simulink model "RTInductionMotorJan27"  (R2020a)
settings: Solver=FixedStepAuto  StartTime=0.0  StopTime=5  FixedStep=100e-6  RelTol=1e-3
model workspace (MAT data in the model file):
  Fe = 60
  Poles = 2
libraries: powerlib x26, simulink x4, powerlib_meascontrol x4
(part 1 of 2)
settings Model: Creator=adam_  LastModifiedBy=Yaipiti
settings SolverCC: AlgebraicLoopSolver=LineSearch
settings SFSimCC: CustomCodeUndefinedFunction=UseInterfaceOnly

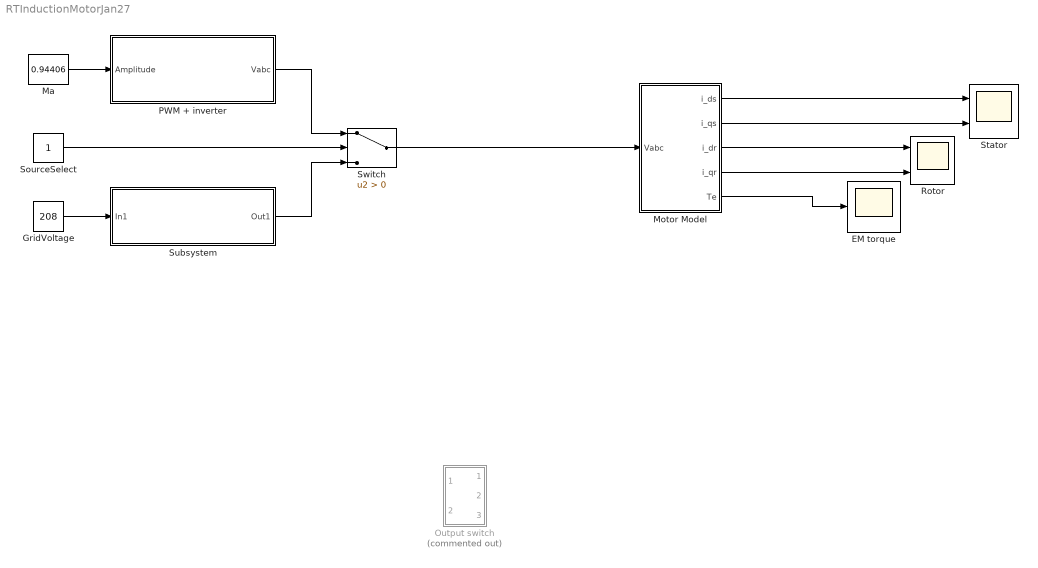
== system RTInductionMotorJan27 ==
  EM torque : Scope
  GridVoltage : Constant  Value=208
  Ma : Constant  Value=0.94406
  Motor Model : Subsystem
  Output switch : Subsystem  Commented=on
  PWM + inverter : Subsystem
  Rotor : Scope  NumInputPorts=2
  SourceSelect : Constant
  Stator : Scope  NumInputPorts=2
  Subsystem : Subsystem
  Switch : Switch  Criteria=u2 > Threshold
  wires:
  Motor Model/1(i_ds) -> Stator/1
  Motor Model/2(i_qs) -> Stator/2
  Motor Model/3(i_dr) -> Rotor/1
  Motor Model/4(i_qr) -> Rotor/2
  Motor Model/5(Te) -> EM torque/1
  Ma/1 -> PWM + inverter/1(Amplitude)
  GridVoltage/1 -> Subsystem/1(In1)
  Subsystem/1(Out1) -> Switch/3
  Switch/1 -> Motor Model/1(Vabc)
  SourceSelect/1 -> Switch/2
  PWM + inverter/1(Vabc) -> Switch/1

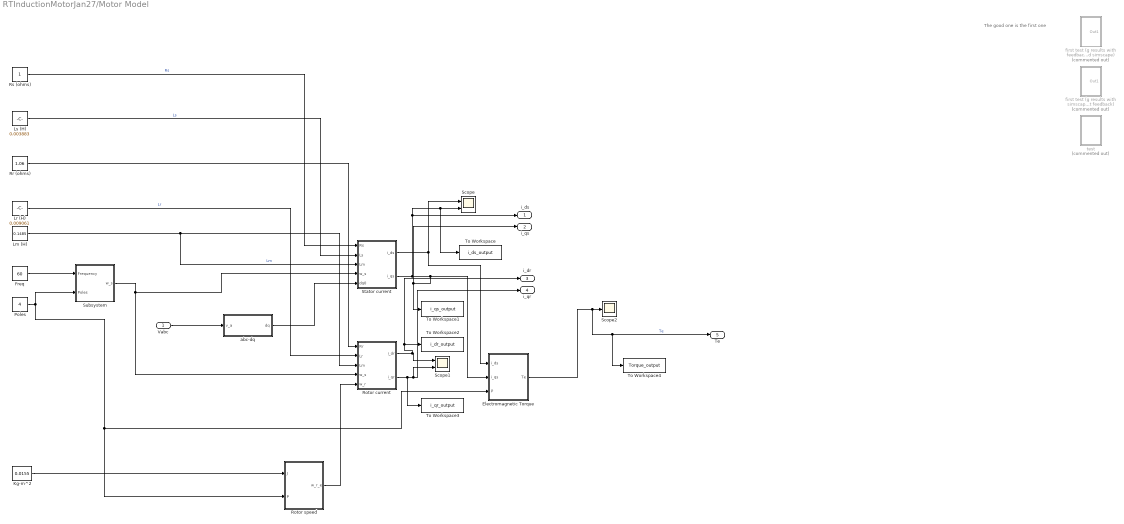
== system RTInductionMotorJan27/Motor Model ==
  note: The good one is the first one
  Vabc : Inport
  Electromagnetic Torque : Subsystem
  Freq : Constant  Value=60
  Kg-m^2 : Constant  Value=0.0155
  Lm (H) : Constant  Value=0.1485
  Lr (H) : Constant  Value=0.009061
  Ls (H) : Constant  Value=0.003883
  Poles : Constant  Value=4
  Rotor current : Subsystem
  Rotor speed : Subsystem
  Rr (ohms) : Constant  Value=1.06
  Rs (ohms) : Constant
  Scope : Scope  NumInputPorts=2
  Scope1 : Scope  NumInputPorts=2
  Scope2 : Scope
  Stator current : Subsystem
  Subsystem : Subsystem
  To Workspace : ToWorkspace  VariableName=i_ds_output  SaveFormat=Timeseries  SampleTime=-1
  To Workspace1 : ToWorkspace  VariableName=i_qs_output  SaveFormat=Timeseries  SampleTime=-1
  To Workspace2 : ToWorkspace  VariableName=i_dr_output  SaveFormat=Timeseries  SampleTime=-1
  To Workspace3 : ToWorkspace  VariableName=i_qr_output  SaveFormat=Timeseries  SampleTime=-1
  To Workspace4 : ToWorkspace  VariableName=Torque_output  SaveFormat=Timeseries  SampleTime=-1
  abc-dq : Subsystem
  first test (g results with feedback and simscape) : Subsystem  Commented=on
  first test (g results with simscape but without feedback) : Subsystem  Commented=on
  test : Subsystem  Commented=on
  i_ds : Outport
  i_qs : Outport  Port=2
  i_dr : Outport  Port=3
  i_qr : Outport  Port=4
  Te : Outport  Port=5
  wires:
  Vabc/1 -> abc-dq/1(v_a)
  Electromagnetic Torque/1(Te) -> Te/1, To Workspace4/1, Scope2/1  "Te"
  Lm (H)/1 -> Rotor current/3(Lm), Stator current/3(Lm)  "Lm"
  abc-dq/1(dq) -> Stator current/5(dq0)
  Lr (H)/1 -> Rotor current/2(Lr)  "Lr"
  Rs (ohms)/1 -> Stator current/1(Rs)  "Rs"
  Subsystem/1(w_s) -> Rotor current/4(w_s), Stator current/4(w_s)
  Kg-m^2/1 -> Rotor speed/1(J)
  Ls (H)/1 -> Stator current/2(Ls)  "Ls"
  Stator current/1(i_ds) -> Electromagnetic Torque/1(i_ds), Scope/1
  Freq/1 -> Subsystem/1(Frequency)
  Rotor speed/1(w_r_e) -> Rotor current/5(w_r)
  Rr (ohms)/1 -> Rotor current/1(Rr)
  Stator current/2(i_qs) -> To Workspace1/1, i_qs/1, Electromagnetic Torque/2(i_qs), i_ds/1, To Workspace/1, Scope/2
  Rotor current/2(i_qr) -> To Workspace3/1, i_qr/1, Scope1/2
  Poles/1 -> Subsystem/2(Poles), Rotor speed/2(P), Electromagnetic Torque/3(P)
  Rotor current/1(i_dr) -> i_dr/1, To Workspace2/1, Scope1/1

== system RTInductionMotorJan27/Output switch ==
  Signal : Inport
  Choice : Inport  Port=2
  Add : Sum  Inputs=+-
  Add1 : Sum  Inputs=+-
  Add2 : Sum  Inputs=+-
  Constant1 : Constant  Value=2
  Constant2 : Constant
  Constant3 : Constant  Value=3
  IsZero : simulink/Logic and Bit Operations/Compare To Zero  relop===  OutDataTypeStr=boolean
  IsZero1 : simulink/Logic and Bit Operations/Compare To Zero  relop===  OutDataTypeStr=boolean
  IsZero2 : simulink/Logic and Bit Operations/Compare To Zero  relop===  OutDataTypeStr=boolean
  Product : Product
  Product1 : Product
  Product2 : Product
  Out1 : Outport
  Out2 : Outport  Port=2
  Out3 : Outport  Port=3
  wires:
  Add1/1 -> IsZero1/1
  Product2/1 -> Out3/1
  Signal/1 -> Product/2, Product1/2, Product2/2
  Choice/1 -> Add2/1, Add1/1, Add/1
  IsZero2/1 -> Product2/1
  Constant1/1 -> Add/2
  Add/1 -> IsZero/1
  Add2/1 -> IsZero2/1
  Constant3/1 -> Add2/2
  IsZero/1 -> Product/1
  Constant2/1 -> Add1/2
  IsZero1/1 -> Product1/1
  Product1/1 -> Out2/1
  Product/1 -> Out1/1

== system RTInductionMotorJan27/PWM + inverter ==
  Amplitude : Inport
  Mux : Mux  Inputs=3
  Product : Product
  Product1 : Product
  Product2 : Product
  Scope : Scope
  Sine Wave : Sin  Frequency=2*pi*60  SampleTime=0
  Sine Wave1 : Sin  Frequency=2*pi*60  Phase=-2*pi/3  SampleTime=0
  Sine Wave2 : Sin  Frequency=2*pi*60  Phase=2*pi/3  SampleTime=0
  Three-phase PWM : Subsystem
  Vdc : Constant  Value=360
  inverter : Subsystem
  Vabc : Outport
  wires:
  Mux/1 -> Three-phase PWM/1(Signals)
  Three-phase PWM/1(Pulses) -> inverter/2(Pulses)
  inverter/1(Vabc) -> Scope/1, Vabc/1
  Vdc/1 -> inverter/1(Vdc)
  Sine Wave/1 -> Product/2
  Amplitude/1 -> Product2/1, Product1/1, Product/1
  Product/1 -> Mux/1
  Product2/1 -> Mux/3
  Product1/1 -> Mux/2
  Sine Wave1/1 -> Product1/2
  Sine Wave2/1 -> Product2/2

== system RTInductionMotorJan27/Subsystem ==
  In1 : Inport
  Mux : Mux  Inputs=3
  Product : Product
  Product1 : Product
  Product2 : Product
  Sine Wave : Sin  Frequency=2*pi*60  SampleTime=0
  Sine Wave1 : Sin  Frequency=2*pi*60  Phase=-2*pi/3  SampleTime=0
  Sine Wave2 : Sin  Frequency=2*pi*60  Phase=2*pi/3  SampleTime=0
  Out1 : Outport
  wires:
  Sine Wave/1 -> Product/2
  Product/1 -> Mux/1
  In1/1 -> Product2/1, Product1/1, Product/1
  Sine Wave1/1 -> Product1/2
  Sine Wave2/1 -> Product2/2
  Product2/1 -> Mux/3
  Product1/1 -> Mux/2
  Mux/1 -> Out1/1

== system RTInductionMotorJan27/Motor Model/Electromagnetic Torque ==
  i_ds : Inport
  i_qs : Inport  Port=2
  P : Inport  Port=3
  Constant : Constant  Value=3/4
  Product{,1..3} (4 alike) : Product
  Subtract : Sum  Inputs=+-
  Te : Outport  VectorParamsAs1DForOutWhenUnconnected=off
  tag scope: Te=global
  wires:
  Product3/1 -> Te/1, [Te]
  Subtract/1 -> Product3/1
  Product2/1 -> Product3/2
  Constant/1 -> Product2/2
  P/1 -> Product2/1
  Product1/1 -> Subtract/2
  Product/1 -> Subtract/1
  i_ds/1 -> Product1/2
  [flux_qs] -> Product1/1
  [flux_ds] -> Product/2
  i_qs/1 -> Product/1

== system RTInductionMotorJan27/Motor Model/Rotor current ==
  Rr : Inport
  Lr : Inport  Port=2
  Lm : Inport  Port=3
  w_s : Inport  Port=4
  w_r : Inport  Port=5
  Rotor Flux : Subsystem
  Rotor currents : Subsystem
  Subtract : Sum  Inputs=+-
  i_dr : Outport  VectorParamsAs1DForOutWhenUnconnected=off
  i_qr : Outport  Port=2  VectorParamsAs1DForOutWhenUnconnected=off
  wires:
  Subtract/1 -> Rotor Flux/2(w_s1)
  w_r/1 -> Subtract/2
  Rotor currents/2(i_qr) -> i_qr/1
  Rotor currents/1(i_dr) -> i_dr/1
  Rotor Flux/1(flux_dr) -> Rotor currents/1(flux_dr)  "flux_dr"
  Rotor Flux/2(flux_qr) -> Rotor currents/2(flus_qr)  "flux_qr"
  Lr/1 -> Rotor currents/3(Lr)
  w_s/1 -> Subtract/1
  Rr/1 -> Rotor Flux/1(Rr (Ohms))
  Lm/1 -> Rotor currents/4(Lm)

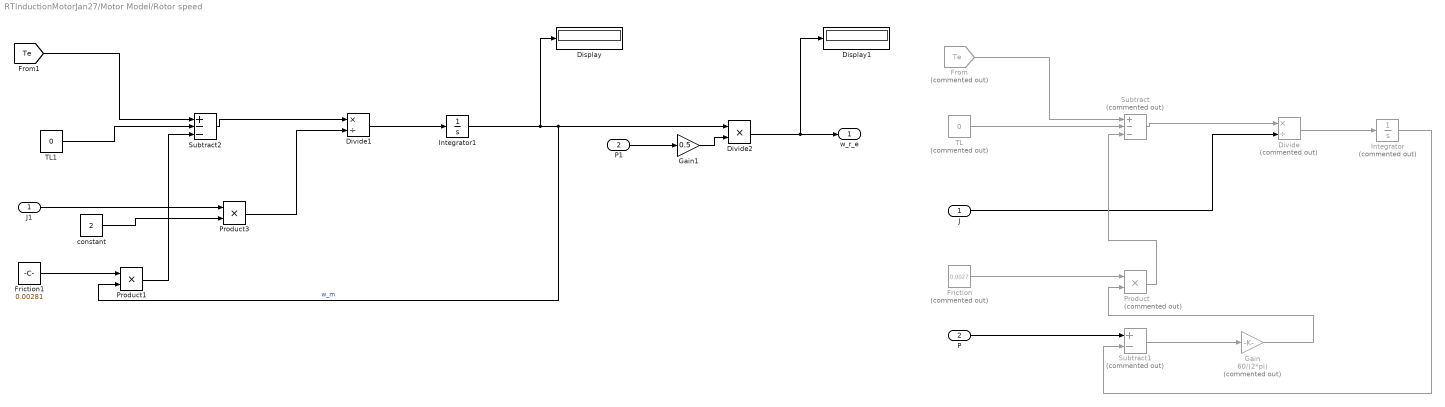
== system RTInductionMotorJan27/Motor Model/Rotor speed ==
  J : Inport
  P : Inport  Port=2
  Display : Display
  Display1 : Display
  Divide : Product  Commented=on  Inputs=*/
  Divide1 : Product  Inputs=*/
  Divide2 : Product  Inputs=**
  Friction : Constant  Commented=on  Value=0.0027
  Friction1 : Constant  Value=0.00281
  From : From  Commented=on  GotoTag=Te  TagVisibility=global
  Gain : Gain  Commented=on  Gain=60/(2*pi)
  Gain1 : Gain  Gain=0.5
  Integrator : Integrator  Commented=on
  Integrator1 : Integrator
  J1 : InportShadow
  P1 : InportShadow  Port=2
  Product : Product  Commented=on
  Product1 : Product
  Product3 : Product
  Subtract : Sum  Commented=on  Inputs=+--
  Subtract1 : Sum  Commented=on  Inputs=+-
  Subtract2 : Sum  Inputs=+--
  TL : Constant  Commented=on  Value=0
  TL1 : Constant  Value=0
  constant : Constant  Value=2
  w_r_e : Outport  VectorParamsAs1DForOutWhenUnconnected=off
  wires:
  From/1 -> Subtract/1
  TL/1 -> Subtract/2
  Subtract/1 -> Divide/1
  J/1 -> Divide/2
  Divide/1 -> Integrator/1
  Integrator/1 -> Subtract1/2
  P/1 -> Subtract1/1
  Subtract1/1 -> Gain/1
  Gain/1 -> Product/2
  Friction/1 -> Product/1
  Product/1 -> Subtract/3
  [Te] -> Subtract2/1
  Subtract2/1 -> Divide1/1
  Divide1/1 -> Integrator1/1
  TL1/1 -> Subtract2/2
  Friction1/1 -> Product1/1
  Product1/1 -> Subtract2/3
  J1/1 -> Product3/1
  constant/1 -> Product3/2
  Product3/1 -> Divide1/2
  Integrator1/1 -> Display/1, Product1/2, Divide2/1  "w_m"
  P1/1 -> Gain1/1
  Gain1/1 -> Divide2/2
  Divide2/1 -> Display1/1, w_r_e/1

== system RTInductionMotorJan27/Motor Model/Stator current ==
  Rs : Inport
  Ls : Inport  Port=2
  Lm : Inport  Port=3
  w_s : Inport  Port=4
  dq0 : Inport  Port=5
  Stator Flux : Subsystem
  Stator currents : Subsystem
  i_ds : Outport  VectorParamsAs1DForOutWhenUnconnected=off
  i_qs : Outport  Port=2  VectorParamsAs1DForOutWhenUnconnected=off
  wires:
  dq0/1 -> Stator Flux/3(dq0)
  Stator currents/2(i_qs) -> i_qs/1
  w_s/1 -> Stator Flux/2(w_s)
  Stator currents/1(i_ds) -> i_ds/1
  Lm/1 -> Stator currents/4(Lm)
  Ls/1 -> Stator currents/3(Ls)
  Rs/1 -> Stator Flux/1(Rs (Ohms))
  Stator Flux/1(flux_ds) -> Stator currents/1(flus_ds)  "flux_ds"
  Stator Flux/2(flux_qs) -> Stator currents/2(flus_qs)  "flux_qs"

== system RTInductionMotorJan27/Motor Model/Subsystem ==
  Frequency : Inport
  Poles : Inport  Port=2
  Constant : Constant  Commented=on  Value=120
  Constant1 : Constant  Commented=on  Value=2*pi
  Display : Display
  Divide2 : Product  Inputs=**/
  Frequency1 : InportShadow
  Gain : Gain  Gain=0.5
  Integrator : Integrator  Commented=on
  Poles1 : InportShadow  Port=2
  Product : Product
  Rem : Math  Commented=on  Operator=rem  SignedPower=on  SaturateOnIntegerOverflow=on
  constant1 : Constant  Value=120
  multipliy : Product  Commented=on  Inputs=**
  ns (rpm) : Product  Commented=on  Inputs=**/
  rpm to rad/s : Gain  Gain=2*pi/60
  w_s_gain : Gain  Commented=on  Gain=2*pi/60
  w_s : Outport  VectorParamsAs1DForOutWhenUnconnected=off
  wires:
  Integrator/1 -> Rem/1
  Rem/1 -> ?
  Constant1/1 -> Rem/2
  Constant/1 -> ns (rpm)/2
  Frequency/1 -> ns (rpm)/1
  Poles/1 -> multipliy/2, ns (rpm)/3
  ns (rpm)/1 -> multipliy/1
  w_s_gain/1 -> Integrator/1  "w_s"
  multipliy/1 -> w_s_gain/1
  constant1/1 -> Divide2/1
  Divide2/1 -> rpm to rad/s/1  "n_s"
  Frequency1/1 -> Divide2/2
  Poles1/1 -> Gain/1, Divide2/3
  rpm to rad/s/1 -> Display/1, Product/1
  Product/1 -> w_s/1
  Gain/1 -> Product/2

== system RTInductionMotorJan27/Motor Model/abc-dq ==
  v_a : Inport
  Add : Sum
  Constant : Constant  Value=2*pi*60
  Constant1 : Constant  Value=-pi/3
  Integrator : Integrator
  Mux3 : Mux  Inputs=2
  Mux4 : Mux  Inputs=2
  Scope2 : Scope
  Scope3 : Scope
  Vd : Fcn  Expr=sqrt(2/3)*(u(1)*cos(u(4))+u(2)*cos(u(4)-2*pi/3)+u(3)*cos(u(4)+2*pi/3))
  Vq : Fcn  Expr=-sqrt(2/3)*(u(1)*sin(u(4))+u(2)*sin(u(4)-2*pi/3)+u(3)*sin(u(4)+2*pi/3))
  dq : Outport  VectorParamsAs1DForOutWhenUnconnected=off
  wires:
  v_a/1 -> Mux3/1
  Mux3/1 -> Vd/1, Vq/1, Scope2/1
  Constant/1 -> Integrator/1
  Integrator/1 -> Add/1  "w_t"
  Constant1/1 -> Add/2
  Add/1 -> Mux3/2
  Vd/1 -> Mux4/1
  Vq/1 -> Mux4/2
  Mux4/1 -> dq/1, Scope3/1

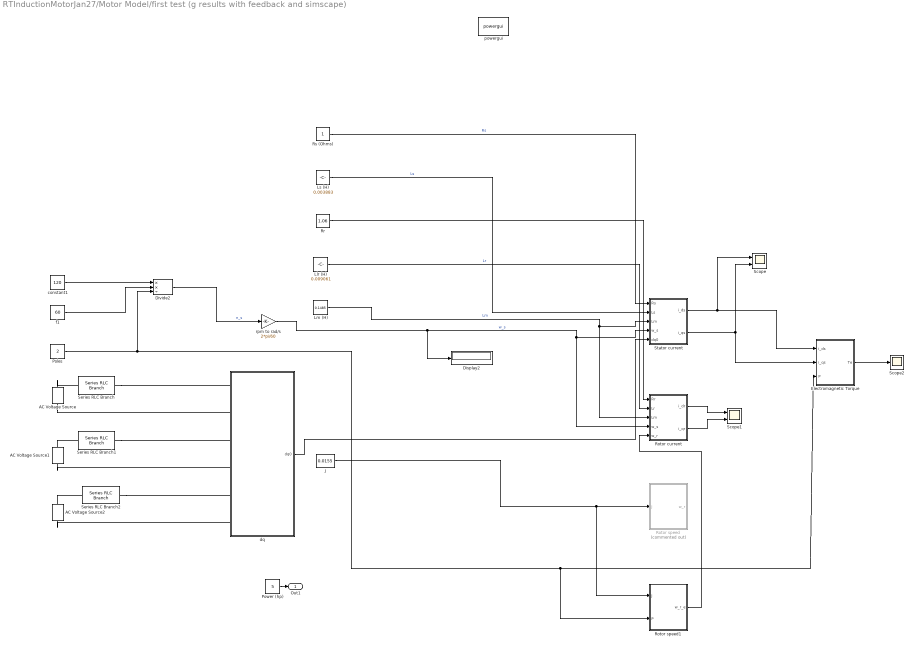
== system RTInductionMotorJan27/Motor Model/first test (g results with feedback and simscape) ==
  AC Voltage Source : powerlib/Electrical Sources/AC Voltage Source  Amplitude=340  Phase=0  Frequency=50  SampleTime=0  Measurements=Voltage  BusType=swing  Pref=10e3  Qref=0  Qmin=-inf  Qmax=+inf
  AC Voltage Source1 : powerlib/Electrical Sources/AC Voltage Source  Amplitude=340  Phase=-120  Frequency=50  SampleTime=0  Measurements=Voltage  BusType=swing  Pref=10e3  Qref=0  Qmin=-inf  Qmax=+inf
  AC Voltage Source2 : powerlib/Electrical Sources/AC Voltage Source  Amplitude=340  Phase=120  Frequency=50  SampleTime=0  Measurements=Voltage  BusType=swing  Pref=10e3  Qref=0  Qmin=-inf  Qmax=+inf
  Display2 : Display
  Divide2 : Product  Inputs=**/
  Electromagnetic Torque : Subsystem
  J : Constant  Value=0.0155
  Llr (H) : Constant  Value=0.009061
  Lm (H) : Constant  Value=0.1485
  Ls (H) : Constant  Value=0.003883
  Poles : Constant  Value=2
  Power (hp) : Constant  Value=5
  Rotor current : Subsystem
  Rotor speed : Subsystem  Commented=on
  Rotor speed1 : Subsystem
  "Rr " : Constant  Value=1.06
  Rs (Ohms) : Constant
  Scope : Scope  NumInputPorts=2
  Scope1 : Scope  NumInputPorts=2
  Scope2 : Scope
  Series RLC Branch : powerlib/Elements/Series RLC Branch  LConnTagsString=__new0  RConnTagsString=__new0  BranchType=R  Resistance=0.1  Inductance=1e-3  SetiL0=off  InitialCurrent=0  Capacitance=1e-6  Setx0=off  InitialVoltage=0  Measurements=None
  Series RLC Branch1 : powerlib/Elements/Series RLC Branch  LConnTagsString=__new0  RConnTagsString=__new0  BranchType=R  Resistance=0.1  Inductance=1e-3  SetiL0=off  InitialCurrent=0  Capacitance=1e-6  Setx0=off  InitialVoltage=0  Measurements=None
  Series RLC Branch2 : powerlib/Elements/Series RLC Branch  LConnTagsString=__new0  RConnTagsString=__new0  BranchType=R  Resistance=0.1  Inductance=1e-3  SetiL0=off  InitialCurrent=0  Capacitance=1e-6  Setx0=off  InitialVoltage=0  Measurements=None
  Stator current : Subsystem
  constant1 : Constant  Value=120
  dq : Subsystem
  f1 : Constant  Value=60
  powergui : powerlib/powergui  Priority=1  SimulationMode=Continuous  SampleTime=50e-6  frequency=60  Iterations=50  frequencyindice=50  Pbase=100e6  ErrMax=1e-4  UnitsV=kV  UnitsW=MW  buscounter=0  FunctionMessages=off  echomessages=off  EnableUseOfTLC=off  CurrentSourceSwitches=off  DisableSnubberDevices=off  DisableRonSwitches=off  DisableVfSwitches=off  DisplayEquations=off  AutomaticDiscreteSolvers=off  SolverType=Tustin/Backward Euler (TBE)  Interpol=off  ExternalGateDelay=off  methode=off  Ts=100  x0status=blocks  SPID=on  SwTol=0  HookPort=off  NonlinearTolerance=1e-4  nMaxIteration=100  ContinueOnMaxIteration=off  RestoreLinks=warning  ResistiveCurrentMeasurement=off  Frange=[0:2:500]  Ylog=off  Xlog=on  ShowGrid=off  save=off  variable=ZData  structure=0  ZoomFFT=off  StartTime=0.0  cycles=1  DisplayStyle=1  fundamental=60  FreqAxis=off  MaxFrequency=1000  frequencyindicesteady=1  RmsSteady=1  display=off
  rpm to rad/s : Gain  Gain=2*pi/60
  Out1 : Outport  VectorParamsAs1DForOutWhenUnconnected=off
  wires:
  J/1 -> Rotor speed1/1(J), Rotor speed/1(J)
  Stator current/2(i_qs) -> Scope/2, Electromagnetic Torque/2(i_qs)
  Electromagnetic Torque/1(Te) -> Scope2/1
  Rotor current/2(i_qr) -> Scope1/2
  "Rr "/1 -> Rotor current/1(Rr)
  Ls (H)/1 -> Stator current/2(Ls)  "Ls"
  rpm to rad/s/1 -> Display2/1, Rotor current/4(w_s), Stator current/4(w_s)  "w_s"
  Lm (H)/1 -> Rotor current/3(Lm), Stator current/3(Lm)  "Lm"
  Poles/1 -> Divide2/3, Rotor speed1/2(P), Electromagnetic Torque/3(P)
  Rotor current/1(i_dr) -> Scope1/1
  Stator current/1(i_ds) -> Scope/1, Electromagnetic Torque/1(i_ds)
  Llr (H)/1 -> Rotor current/2(Lr)  "Lr"
  Rs (Ohms)/1 -> Stator current/1(Rs)  "Rs"
  dq/1(dq0) -> Stator current/5(dq0)
  Power (hp)/1 -> Out1/1
  Rotor speed1/1(w_r_e) -> Rotor current/5(w_r)
  f1/1 -> Divide2/2
  constant1/1 -> Divide2/1
  Divide2/1 -> rpm to rad/s/1  "n_s"
  connections:
  AC Voltage Source/LConn1 -- dq/LConn2
  Series RLC Branch2/RConn1 -- dq/LConn5
  AC Voltage Source2/RConn1 -- Series RLC Branch2/LConn1
  AC Voltage Source1/RConn1 -- Series RLC Branch1/LConn1
  AC Voltage Source/RConn1 -- Series RLC Branch/LConn1
  AC Voltage Source2/LConn1 -- dq/LConn6
  Series RLC Branch/RConn1 -- dq/LConn1
  AC Voltage Source1/LConn1 -- dq/LConn4
  Series RLC Branch1/RConn1 -- dq/LConn3

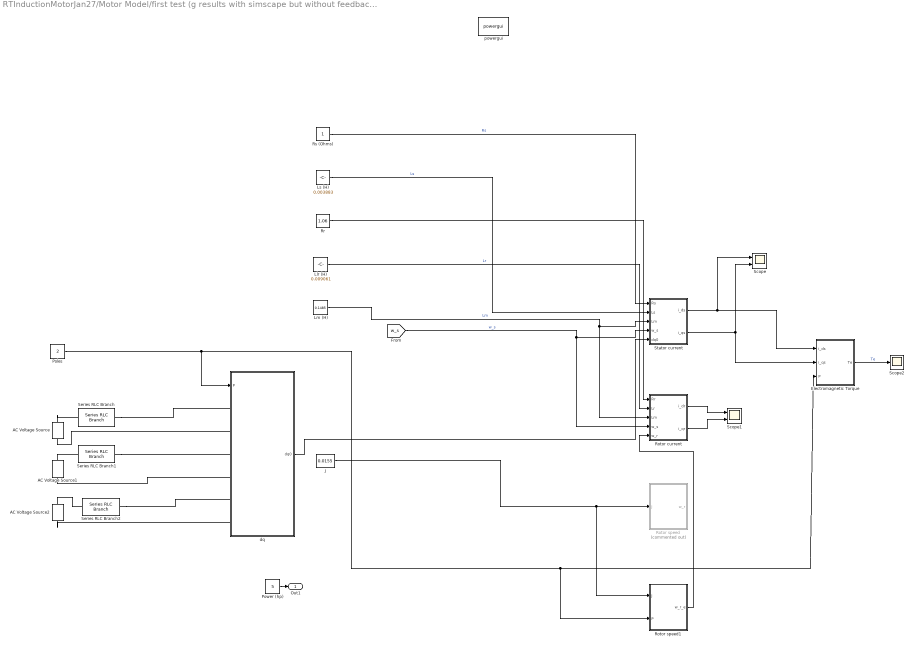
== system RTInductionMotorJan27/Motor Model/first test (g results with simscape but without feedback) ==
  AC Voltage Source : powerlib/Electrical Sources/AC Voltage Source  Amplitude=340  Phase=0  Frequency=50  SampleTime=0  Measurements=None  BusType=swing  Pref=10e3  Qref=0  Qmin=-inf  Qmax=+inf
  AC Voltage Source1 : powerlib/Electrical Sources/AC Voltage Source  Amplitude=340  Phase=-120  Frequency=50  SampleTime=0  Measurements=None  BusType=swing  Pref=10e3  Qref=0  Qmin=-inf  Qmax=+inf
  AC Voltage Source2 : powerlib/Electrical Sources/AC Voltage Source  Amplitude=340  Phase=120  Frequency=50  SampleTime=0  Measurements=None  BusType=swing  Pref=10e3  Qref=0  Qmin=-inf  Qmax=+inf
  Electromagnetic Torque : Subsystem
  J : Constant  Value=0.0155
  Llr (H) : Constant  Value=0.009061
  Lm (H) : Constant  Value=0.1485
  Ls (H) : Constant  Value=0.003883
  Poles : Constant  Value=2
  Power (hp) : Constant  Value=5
  Rotor current : Subsystem
  Rotor speed : Subsystem  Commented=on
  Rotor speed1 : Subsystem
  "Rr " : Constant  Value=1.06
  Rs (Ohms) : Constant
  Scope : Scope  NumInputPorts=2
  Scope1 : Scope  NumInputPorts=2
  Scope2 : Scope
  Series RLC Branch : powerlib/Elements/Series RLC Branch  LConnTagsString=__new0  RConnTagsString=__new0  BranchType=R  Resistance=0.1  Inductance=1e-3  SetiL0=off  InitialCurrent=0  Capacitance=1e-6  Setx0=off  InitialVoltage=0  Measurements=None
  Series RLC Branch1 : powerlib/Elements/Series RLC Branch  LConnTagsString=__new0  RConnTagsString=__new0  BranchType=R  Resistance=0.1  Inductance=1e-3  SetiL0=off  InitialCurrent=0  Capacitance=1e-6  Setx0=off  InitialVoltage=0  Measurements=None
  Series RLC Branch2 : powerlib/Elements/Series RLC Branch  LConnTagsString=__new0  RConnTagsString=__new0  BranchType=R  Resistance=0.1  Inductance=1e-3  SetiL0=off  InitialCurrent=0  Capacitance=1e-6  Setx0=off  InitialVoltage=0  Measurements=None
  Stator current : Subsystem
  dq : Subsystem
  powergui : powerlib/powergui  Priority=1  SimulationMode=Continuous  SampleTime=50e-6  frequency=60  Iterations=50  frequencyindice=50  Pbase=100e6  ErrMax=1e-4  UnitsV=kV  UnitsW=MW  buscounter=0  FunctionMessages=off  echomessages=off  EnableUseOfTLC=off  CurrentSourceSwitches=off  DisableSnubberDevices=off  DisableRonSwitches=off  DisableVfSwitches=off  DisplayEquations=off  AutomaticDiscreteSolvers=off  SolverType=Tustin/Backward Euler (TBE)  Interpol=off  ExternalGateDelay=off  methode=off  Ts=100  x0status=blocks  SPID=on  SwTol=0  HookPort=off  NonlinearTolerance=1e-4  nMaxIteration=100  ContinueOnMaxIteration=off  RestoreLinks=warning  ResistiveCurrentMeasurement=off  Frange=[0:2:500]  Ylog=off  Xlog=on  ShowGrid=off  save=off  variable=ZData  structure=0  ZoomFFT=off  StartTime=0.0  cycles=1  DisplayStyle=1  fundamental=60  FreqAxis=off  MaxFrequency=1000  frequencyindicesteady=1  RmsSteady=1  display=off
  Out1 : Outport  VectorParamsAs1DForOutWhenUnconnected=off
  wires:
  Rotor speed1/1(w_r_e) -> Rotor current/5(w_r)
  Power (hp)/1 -> Out1/1
  dq/1(dq0) -> Stator current/5(dq0)
  Rs (Ohms)/1 -> Stator current/1(Rs)  "Rs"
  Llr (H)/1 -> Rotor current/2(Lr)  "Lr"
  Stator current/1(i_ds) -> Electromagnetic Torque/1(i_ds), Scope/1
  Rotor current/1(i_dr) -> Scope1/1
  Poles/1 -> Electromagnetic Torque/3(P), Rotor speed1/2(P), dq/1(P)
  Lm (H)/1 -> Stator current/3(Lm), Rotor current/3(Lm)  "Lm"
  [w_s] -> Stator current/4(w_s), Rotor current/4(w_s)  "w_s"
  Ls (H)/1 -> Stator current/2(Ls)  "Ls"
  "Rr "/1 -> Rotor current/1(Rr)
  Rotor current/2(i_qr) -> Scope1/2
  Electromagnetic Torque/1(Te) -> Scope2/1  "Te"
  Stator current/2(i_qs) -> Electromagnetic Torque/2(i_qs), Scope/2
  J/1 -> Rotor speed/1(J), Rotor speed1/1(J)
  connections:
  Series RLC Branch1/RConn1 -- dq/LConn3
  AC Voltage Source1/LConn1 -- dq/LConn4
  Series RLC Branch/RConn1 -- dq/LConn1
  AC Voltage Source2/LConn1 -- dq/LConn6
  AC Voltage Source/RConn1 -- Series RLC Branch/LConn1
  AC Voltage Source1/RConn1 -- Series RLC Branch1/LConn1
  AC Voltage Source2/RConn1 -- Series RLC Branch2/LConn1
  Series RLC Branch2/RConn1 -- dq/LConn5
  AC Voltage Source/LConn1 -- dq/LConn2

== system RTInductionMotorJan27/Motor Model/test ==
  Asynchronous Machine pu Units : powerlib/Machines/Asynchronous Machine pu Units  Commented=on  RotorType=Squirrel-cage  PresetModel=No  MechanicalLoad=Torque Tm  ShowDetailedParameters=on  ReferenceFrame=Rotor  Units=pu  MeasurementBus=off  NominalParameters=[3730 460 60]  Stator=[0.01965 0.0397]  Rotor=[0.01909 0.0397]  Cage1=[0.01909 0.0397]  Cage2=[0.01909 0.0397]  Lm=1.354  Mechanical=[0.09526 0.05479 2]  PolePairs=2  InitialConditions="[ 1,0   0,0,0   0,0,0 ]"  SimulateSaturation=off  Saturation="[0.212,0.4201,0.8125,1.0979,1.4799,2.2457,3.2586,4.5763,6.4763 ;   0.5,0.7,0.9,1,1.1,1.2 ,1.3,1.4,1.5]"  LoadFlowParameters=0  TsPowergui=0  TsBlock=-1  IterativeModel=Trapezoidal non iterative  IterativeDiscreteModel=Trapezoidal non iterative  Pmec=0
      settings: SourceProductBaseCode=PS
  Frictional Torque Constant (Nms) : Constant  Value=0.0027
  Induction Machine : Subsystem
  Induction Motor Parameters1 : Subsystem
  Induction Motor Parameters2 : Subsystem  Commented=on
  Scope : Scope
  TL (Nm) : Constant  Value=0
  powergui : powerlib/powergui  Priority=1  SimulationMode=Continuous  SampleTime=50e-6  frequency=60  Iterations=50  frequencyindice=50  Pbase=100e6  ErrMax=1e-4  UnitsV=kV  UnitsW=MW  buscounter=0  FunctionMessages=off  echomessages=off  EnableUseOfTLC=off  CurrentSourceSwitches=off  DisableSnubberDevices=off  DisableRonSwitches=off  DisableVfSwitches=off  DisplayEquations=off  AutomaticDiscreteSolvers=off  SolverType=Tustin/Backward Euler (TBE)  Interpol=off  ExternalGateDelay=off  methode=off  Ts=100  x0status=blocks  SPID=on  SwTol=0  HookPort=off  NonlinearTolerance=1e-4  nMaxIteration=100  ContinueOnMaxIteration=off  RestoreLinks=warning  ResistiveCurrentMeasurement=off  Frange=[0:2:500]  Ylog=off  Xlog=on  ShowGrid=off  save=off  variable=ZData  structure=0  ZoomFFT=off  StartTime=0.0  cycles=1  DisplayStyle=1  fundamental=60  FreqAxis=off  MaxFrequency=1000  frequencyindicesteady=1  RmsSteady=1  display=off
  powergui1 : powerlib/powergui  Priority=1  Commented=on  SimulationMode=Continuous  SampleTime=50e-6  frequency=60  Iterations=50  frequencyindice=50  Pbase=100e6  ErrMax=1e-4  UnitsV=kV  UnitsW=MW  buscounter=0  FunctionMessages=off  echomessages=off  EnableUseOfTLC=off  CurrentSourceSwitches=off  DisableSnubberDevices=off  DisableRonSwitches=off  DisableVfSwitches=off  DisplayEquations=off  AutomaticDiscreteSolvers=off  SolverType=Tustin/Backward Euler (TBE)  Interpol=off  ExternalGateDelay=off  methode=off  Ts=100  x0status=blocks  SPID=on  SwTol=0  HookPort=off  NonlinearTolerance=1e-4  nMaxIteration=100  ContinueOnMaxIteration=off  RestoreLinks=warning  ResistiveCurrentMeasurement=off  Frange=[0:2:500]  Ylog=off  Xlog=on  ShowGrid=off  save=off  variable=ZData  structure=0  ZoomFFT=off  StartTime=0.0  cycles=1  DisplayStyle=1  fundamental=60  FreqAxis=off  MaxFrequency=1000  frequencyindicesteady=1  RmsSteady=1  display=off
  wires:
  Frictional Torque Constant (Nms)/1 -> Induction Machine/3(Frictional Torque (N.m.s))
  TL (Nm)/1 -> Induction Machine/2(TL (Nm))
  Induction Machine/1(EM Torque (Nm)) -> Scope/1  "EM Torque (Nm)"
  Induction Motor Parameters1/1(Induction Motor Paramaters) -> Induction Machine/1(Motor Parameters)

== system RTInductionMotorJan27/PWM + inverter/Three-phase PWM ==
  Signals : Inport
  Constant : Constant  Value=0
  Constant1 : Constant
  Demux : Demux  Outputs=3
  Mux : Mux  Inputs=3
  Output Scope : Scope  NumInputPorts=3
  Scope : Scope  NumInputPorts=4
  Sum : Sum  Inputs=|-+
  Sum1 : Sum  Inputs=|-+
  Sum2 : Sum  Inputs=|-+
  Switch : Switch  Criteria=u2 > Threshold
  Switch1 : Switch  Criteria=u2 > Threshold
  Switch2 : Switch  Criteria=u2 > Threshold
  Triangle Generator : powerlib_meascontrol/Pulse & Signal Generators/Triangle Generator  Freq=27*60  Phase=90  Ts=100e-6
  Pulses : Outport
  wires:
  Sum/1 -> Switch/2
  Triangle Generator/1 -> Scope/4, Sum2/2, Sum1/2, Sum/2
  Constant/1 -> Switch2/1, Switch1/1, Switch/1
  Switch1/1 -> Output Scope/2, Mux/2
  Demux/2 -> Scope/2, Sum1/1
  Switch2/1 -> Output Scope/3, Mux/3
  Constant1/1 -> Switch1/3, Switch/3, Switch2/3
  Switch/1 -> Output Scope/1, Mux/1
  Demux/3 -> Scope/3, Sum2/1
  Sum1/1 -> Switch1/2
  Sum2/1 -> Switch2/2
  Mux/1 -> Pulses/1
  Signals/1 -> Demux/1
  Demux/1 -> Scope/1, Sum/1

== system RTInductionMotorJan27/PWM + inverter/inverter ==
  Vdc : Inport
  Pulses : Inport  Port=2
  Mux : Mux  Inputs=2
  Mux1 : Mux  Inputs=3
  Scope : Scope  NumInputPorts=3
  vaN : Fcn  Expr=u(1)*((2*u(2))-u(3)-u(4))/3
  vbN : Fcn  Expr=u(1)*((2*u(3))-u(2)-u(4))/3
  vcN : Fcn  Expr=u(1)*((2*u(4))-u(3)-u(2))/3
  Vabc : Outport
  wires:
  Vdc/1 -> Mux/1
  Pulses/1 -> Mux/2
  Mux/1 -> vcN/1, vbN/1, vaN/1
  Mux1/1 -> Vabc/1
  vaN/1 -> Scope/1, Mux1/1
  vbN/1 -> Scope/2, Mux1/2
  vcN/1 -> Mux1/3, Scope/3

== system RTInductionMotorJan27/Motor Model/Rotor current/Rotor Flux ==
  Rr (Ohms) : Inport
  w_s1 : Inport  Port=2
  Integrator : Integrator
  Integrator1 : Integrator
  Rr (Ohms)1 : InportShadow
  Subtract : Sum  Inputs=-+
  Subtract1 : Sum  Inputs=--
  product{,1..3} (4 alike) : Product  Inputs=**
  flux_dr : Outport  VectorParamsAs1DForOutWhenUnconnected=off
  flux_qr : Outport  Port=2  VectorParamsAs1DForOutWhenUnconnected=off
  tag scope: flux_dr=global, flux_qr=global
  wires:
  [i_qr] -> product1/2
  product2/1 -> Subtract1/1
  product3/1 -> Subtract/2
  w_s1/1 -> product2/2, product3/1
  Rr (Ohms)1/1 -> product1/1
  Integrator1/1 -> flux_qr/1, [flux_qr], product3/2
  [i_dr] -> product/1
  product1/1 -> Subtract1/2
  Subtract1/1 -> Integrator1/1
  Integrator/1 -> flux_dr/1, [flux_dr], product2/1
  Subtract/1 -> Integrator/1
  product/1 -> Subtract/1
  Rr (Ohms)/1 -> product/2

== system RTInductionMotorJan27/Motor Model/Rotor current/Rotor currents ==
  flux_dr : Inport
  flus_qr : Inport  Port=2
  Lr : Inport  Port=3
  Lm : Inport  Port=4
  Add : Sum
  Divide : Product  Inputs=*/
  Divide1 : Product  Inputs=/*
  Lm1 : InportShadow  Port=4
  Product : Product
  Product1 : Product
  Scope : Scope  NumInputPorts=2
  Subtract : Sum  Inputs=-+
  Subtract1 : Sum  Inputs=-+
  i_dr : Outport  VectorParamsAs1DForOutWhenUnconnected=off
  i_qr : Outport  Port=2  VectorParamsAs1DForOutWhenUnconnected=off
  tag scope: i_dr=global, i_qr=global
  wires:
  Divide1/1 -> i_qr/1, Scope/1, [i_qr]  "i_rs"
  Subtract1/1 -> Divide1/2
  flus_qr/1 -> Subtract1/2
  Product1/1 -> Subtract1/1
  [i_qs] -> Product1/2
  Divide/1 -> i_dr/1, Scope/2, [i_dr]  "i_dr"
  Add/1 -> Divide/2, Divide1/1
  Subtract/1 -> Divide/1
  Lm/1 -> Add/2, Product1/1
  Lr/1 -> Add/1
  Product/1 -> Subtract/1
  flux_dr/1 -> Subtract/2
  [i_ds] -> Product/2
  Lm1/1 -> Product/1

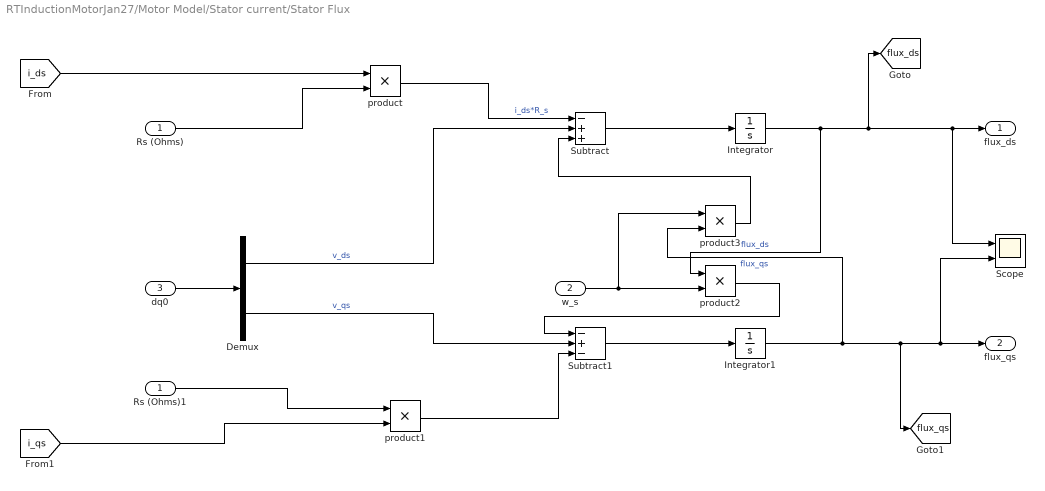
== system RTInductionMotorJan27/Motor Model/Stator current/Stator Flux ==
  Rs (Ohms) : Inport
  w_s : Inport  Port=2
  dq0 : Inport  Port=3
  Demux : Demux  Outputs=2
  Integrator : Integrator
  Integrator1 : Integrator
  Rs (Ohms)1 : InportShadow
  Scope : Scope  NumInputPorts=2
  Subtract : Sum  Inputs=-++
  Subtract1 : Sum  Inputs=-+-
  product{,1..3} (4 alike) : Product  Inputs=**
  flux_ds : Outport  VectorParamsAs1DForOutWhenUnconnected=off
  flux_qs : Outport  Port=2  VectorParamsAs1DForOutWhenUnconnected=off
  tag scope: flux_ds=global, flux_qs=global
  wires:
  Demux/2 -> Subtract1/2  "v_qs"
  Demux/1 -> Subtract/2  "v_ds"
  [i_qs] -> product1/2
  product2/1 -> Subtract1/1
  product3/1 -> Subtract/3
  w_s/1 -> product3/1, product2/2
  Rs (Ohms)1/1 -> product1/1
  Integrator1/1 -> [flux_qs], flux_qs/1, Scope/2, product3/2  "flux_qs"
  [i_ds] -> product/1
  product1/1 -> Subtract1/3
  Subtract1/1 -> Integrator1/1
  Integrator/1 -> [flux_ds], flux_ds/1, Scope/1, product2/1  "flux_ds"
  Subtract/1 -> Integrator/1
  product/1 -> Subtract/1  "i_ds*R_s"
  Rs (Ohms)/1 -> product/2
  dq0/1 -> Demux/1

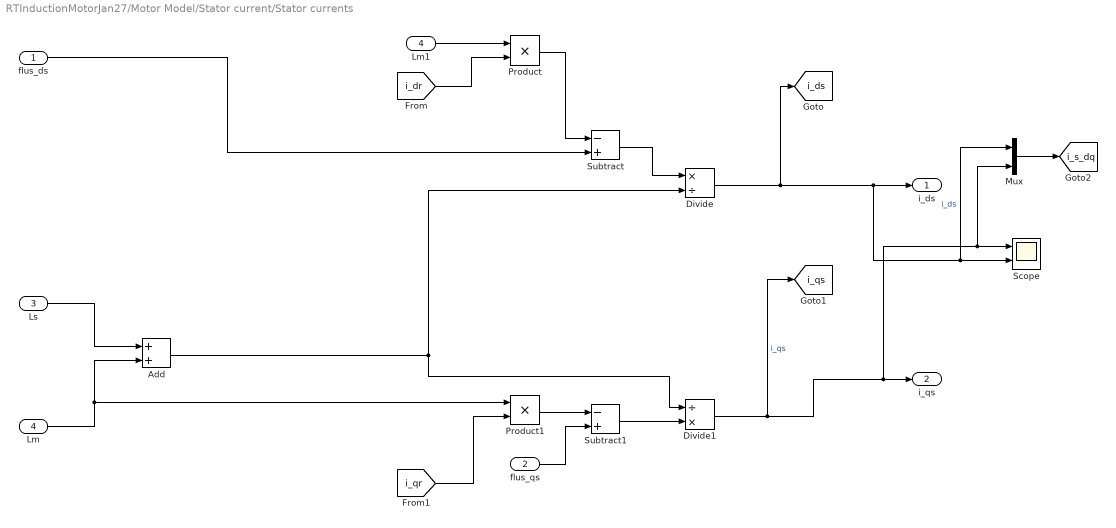
== system RTInductionMotorJan27/Motor Model/Stator current/Stator currents ==
  flus_ds : Inport
  flus_qs : Inport  Port=2
  Ls : Inport  Port=3
  Lm : Inport  Port=4
  Add : Sum
  Divide : Product  Inputs=*/
  Divide1 : Product  Inputs=/*
  Lm1 : InportShadow  Port=4
  Mux : Mux  Inputs=2
  Product : Product
  Product1 : Product
  Scope : Scope  NumInputPorts=2
  Subtract : Sum  Inputs=-+
  Subtract1 : Sum  Inputs=-+
  i_ds : Outport  VectorParamsAs1DForOutWhenUnconnected=off
  i_qs : Outport  Port=2  VectorParamsAs1DForOutWhenUnconnected=off
  tag scope: i_ds=global, i_qs=global, i_s_dq=global
  wires:
  Mux/1 -> [i_s_dq]
  Divide1/1 -> i_qs/1, Scope/1, Mux/2, [i_qs]  "i_qs"
  Subtract1/1 -> Divide1/2
  flus_qs/1 -> Subtract1/2
  Product1/1 -> Subtract1/1
  [i_qr] -> Product1/2
  Divide/1 -> i_ds/1, Scope/2, Mux/1, [i_ds]  "i_ds"
  Add/1 -> Divide/2, Divide1/1
  Subtract/1 -> Divide/1
  Lm/1 -> Add/2, Product1/1
  Ls/1 -> Add/1
  Product/1 -> Subtract/1
  flus_ds/1 -> Subtract/2
  [i_dr] -> Product/2
  Lm1/1 -> Product/1

== system RTInductionMotorJan27/Motor Model/first test (g results with feedback and simscape)/Electromagnetic Torque ==
  i_ds : Inport
  i_qs : Inport  Port=2
  P : Inport  Port=3
  Constant : Constant  Value=3/4
  Product{,1..3} (4 alike) : Product
  Subtract : Sum  Inputs=+-
  Te : Outport  VectorParamsAs1DForOutWhenUnconnected=off
  tag scope: Te=global
  wires:
  i_qs/1 -> Product/1
  [flux_dr] -> Product/2
  [flux_qr] -> Product1/1
  i_ds/1 -> Product1/2
  Product/1 -> Subtract/1
  Product1/1 -> Subtract/2
  Constant/1 -> Product2/2
  Product2/1 -> Product3/2
  Subtract/1 -> Product3/1
  Product3/1 -> [Te], Te/1
  P/1 -> Product2/1

== system RTInductionMotorJan27/Motor Model/first test (g results with feedback and simscape)/Rotor current ==
  Rr : Inport
  Lr : Inport  Port=2
  Lm : Inport  Port=3
  w_s : Inport  Port=4
  w_r : Inport  Port=5
  Rotor Flux : Subsystem
  Rotor currents : Subsystem
  Subtract : Sum  Inputs=+-
  i_dr : Outport  VectorParamsAs1DForOutWhenUnconnected=off
  i_qr : Outport  Port=2  VectorParamsAs1DForOutWhenUnconnected=off
  wires:
  Rotor Flux/2(flux_qr) -> Rotor currents/2(flus_qr)  "flux_qr"
  Rotor Flux/1(flux_dr) -> Rotor currents/1(flux_dr)  "flux_dr"
  Rr/1 -> Rotor Flux/1(Rr (Ohms))
  Lr/1 -> Rotor currents/3(Lr)
  Lm/1 -> Rotor currents/4(Lm)
  Rotor currents/1(i_dr) -> i_dr/1
  Rotor currents/2(i_qr) -> i_qr/1
  w_s/1 -> Subtract/1
  w_r/1 -> Subtract/2
  Subtract/1 -> Rotor Flux/2(w_s1)

== system RTInductionMotorJan27/Motor Model/first test (g results with feedback and simscape)/Rotor speed ==
  J : Inport
  Divide : Product  Inputs=*/
  Integrator : Integrator
  Subtract : Sum  Inputs=+--
  TL : Constant  Value=0
  w_r : Outport  VectorParamsAs1DForOutWhenUnconnected=off
  wires:
  [Te] -> Subtract/1
  TL/1 -> Subtract/2
  Subtract/1 -> Divide/1
  J/1 -> Divide/2
  Divide/1 -> Integrator/1
  Integrator/1 -> Subtract/3, w_r/1

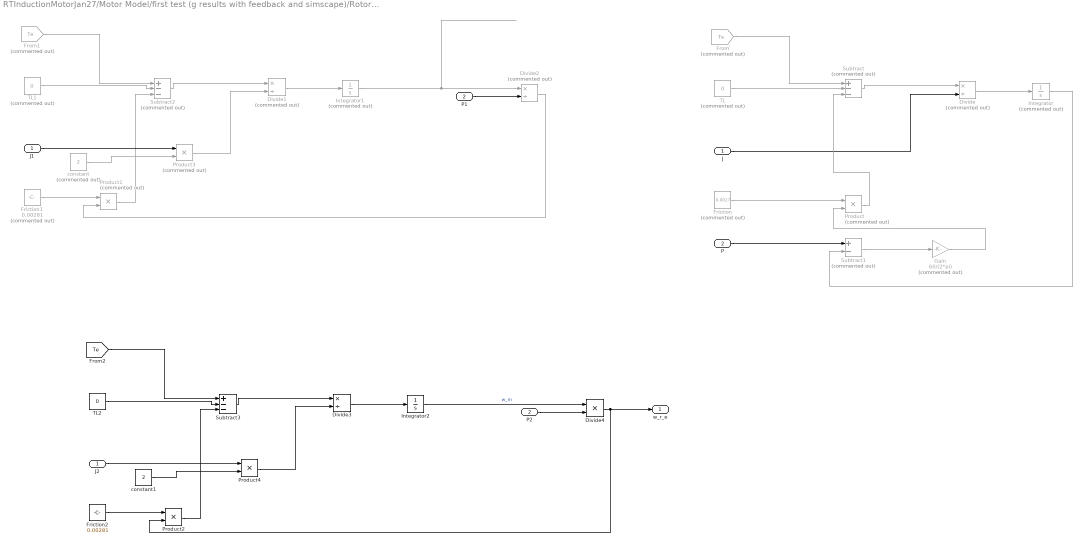
== system RTInductionMotorJan27/Motor Model/first test (g results with feedback and simscape)/Rotor speed1 ==
  J : Inport
  P : Inport  Port=2
  Divide : Product  Commented=on  Inputs=*/
  Divide1 : Product  Commented=on  Inputs=*/
  Divide2 : Product  Commented=on  Inputs=*/
  Divide3 : Product  Inputs=*/
  Divide4 : Product  Inputs=**
  Friction : Constant  Commented=on  Value=0.0027
  Friction1 : Constant  Commented=on  Value=0.00281
  Friction2 : Constant  Value=0.00281
  From : From  Commented=on  GotoTag=Te  TagVisibility=global
  From1 : From  Commented=on  GotoTag=Te  TagVisibility=global
  Gain : Gain  Commented=on  Gain=60/(2*pi)
  Integrator : Integrator  Commented=on
  Integrator1 : Integrator  Commented=on
  Integrator2 : Integrator
  J1 : InportShadow
  J2 : InportShadow
  P1 : InportShadow  Port=2
  P2 : InportShadow  Port=2
  Product : Product  Commented=on
  Product1 : Product  Commented=on
  Product2 : Product
  Product3 : Product  Commented=on
  Product4 : Product
  Subtract : Sum  Commented=on  Inputs=+--
  Subtract1 : Sum  Commented=on  Inputs=+-
  Subtract2 : Sum  Commented=on  Inputs=+--
  Subtract3 : Sum  Inputs=+--
  TL : Constant  Commented=on  Value=0
  TL1 : Constant  Commented=on  Value=0
  TL2 : Constant  Value=0
  constant : Constant  Commented=on  Value=2
  constant1 : Constant  Value=2
  w_r_e : Outport  VectorParamsAs1DForOutWhenUnconnected=off
  wires:
  From/1 -> Subtract/1
  TL/1 -> Subtract/2
  Subtract/1 -> Divide/1
  J/1 -> Divide/2
  Divide/1 -> Integrator/1
  Integrator/1 -> Subtract1/2
  P/1 -> Subtract1/1
  Subtract1/1 -> Gain/1
  Gain/1 -> Product/2
  Friction/1 -> Product/1
  Product/1 -> Subtract/3
  From1/1 -> Subtract2/1
  Subtract2/1 -> Divide1/1
  Divide1/1 -> Integrator1/1
  TL1/1 -> Subtract2/2
  Friction1/1 -> Product1/1
  Product1/1 -> Subtract2/3
  J1/1 -> Product3/1
  constant/1 -> Product3/2
  Product3/1 -> Divide1/2
  Integrator1/1 -> Divide2/1
  P1/1 -> Divide2/2
  Divide2/1 -> Product1/2
  Divide4/1 -> Product2/2, w_r_e/1
  Product2/1 -> Subtract3/3
  J2/1 -> Product4/1
  Subtract3/1 -> Divide3/1
  Integrator2/1 -> Divide4/1  "w_m"
  Divide3/1 -> Integrator2/1
  Friction2/1 -> Product2/1
  Product4/1 -> Divide3/2
  [Te] -> Subtract3/1
  TL2/1 -> Subtract3/2
  constant1/1 -> Product4/2
  P2/1 -> Divide4/2

== system RTInductionMotorJan27/Motor Model/first test (g results with feedback and simscape)/Stator current ==
  Rs : Inport
  Ls : Inport  Port=2
  Lm : Inport  Port=3
  w_s : Inport  Port=4
  dq0 : Inport  Port=5
  Stator Flux : Subsystem
  Stator currents : Subsystem
  i_ds : Outport  VectorParamsAs1DForOutWhenUnconnected=off
  i_qs : Outport  Port=2  VectorParamsAs1DForOutWhenUnconnected=off
  wires:
  Stator Flux/2(flux_qs) -> Stator currents/2(flus_qs)  "flux_qs"
  Stator Flux/1(flux_ds) -> Stator currents/1(flus_ds)  "flux_ds"
  Rs/1 -> Stator Flux/1(Rs (Ohms))
  Ls/1 -> Stator currents/3(Ls)
  Lm/1 -> Stator currents/4(Lm)
  Stator currents/1(i_ds) -> i_ds/1
  w_s/1 -> Stator Flux/2(w_s)
  Stator currents/2(i_qs) -> i_qs/1
  dq0/1 -> Stator Flux/3(dq0)

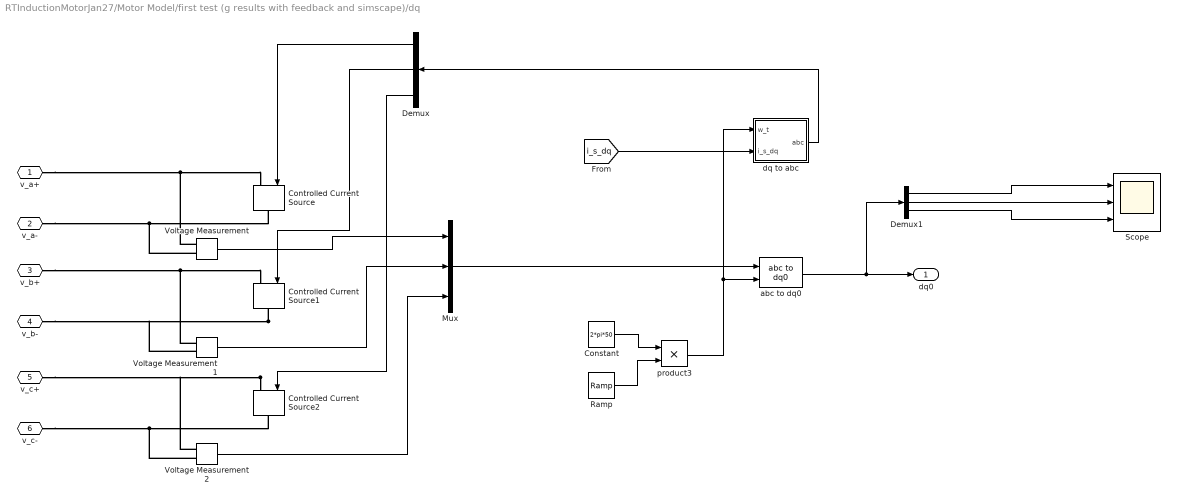
== system RTInductionMotorJan27/Motor Model/first test (g results with feedback and simscape)/dq ==
  Constant : Constant  Value=2*pi*50
  Controlled Current Source : powerlib/Electrical Sources/Controlled Current Source  Initialize=on  Source_Type=AC  Amplitude=0  Phase=0  Frequency=0  Measurements=None
  Controlled Current Source1 : powerlib/Electrical Sources/Controlled Current Source  Initialize=on  Source_Type=AC  Amplitude=0  Phase=0  Frequency=0  Measurements=None
  Controlled Current Source2 : powerlib/Electrical Sources/Controlled Current Source  Initialize=on  Source_Type=AC  Amplitude=0  Phase=0  Frequency=0  Measurements=None
  Demux : Demux  Outputs=3
  Demux1 : Demux  Outputs=3
  Mux : Mux  Inputs=3
  Ramp : simulink/Sources/Ramp  slope=1  start=0  InitialOutput=0
  Scope : Scope  NumInputPorts=3
  Voltage Measurement : powerlib/Measurements/Voltage Measurement  PhasorSimulation=off  OutputType=Complex  PSBequivalent=0
  Voltage Measurement1 : powerlib/Measurements/Voltage Measurement  PhasorSimulation=off  OutputType=Complex  PSBequivalent=0
  Voltage Measurement2 : powerlib/Measurements/Voltage Measurement  PhasorSimulation=off  OutputType=Complex  PSBequivalent=0
  abc to dq0 : powerlib_meascontrol/Transformations/abc to dq0  Alignment=90 degrees behind phase A axis
  dq to abc : Subsystem
  product3 : Product  Inputs=**
  v_a+ : PMIOPort  Side=Left
  v_a- : PMIOPort  Port=2  Side=Left
  v_b+ : PMIOPort  Port=3  Side=Left
  v_b- : PMIOPort  Port=4  Side=Left
  v_c+ : PMIOPort  Port=5  Side=Left
  v_c- : PMIOPort  Port=6  Side=Left
  dq0 : Outport  VectorParamsAs1DForOutWhenUnconnected=off
  wires:
  Voltage Measurement/1 -> Mux/1
  Voltage Measurement1/1 -> Mux/2
  Voltage Measurement2/1 -> Mux/3
  Mux/1 -> abc to dq0/1
  abc to dq0/1 -> Demux1/1, dq0/1
  [i_s_dq] -> dq to abc/2(i_s_dq)
  dq to abc/1(abc) -> Demux/1
  Demux/1 -> Controlled Current Source/1
  Demux/2 -> Controlled Current Source1/1
  Demux/3 -> Controlled Current Source2/1
  Demux1/1 -> Scope/1
  Demux1/2 -> Scope/2
  Demux1/3 -> Scope/3
  Constant/1 -> product3/1
  Ramp/1 -> product3/2
  product3/1 -> dq to abc/1(w_t), abc to dq0/2
  connections:
  Voltage Measurement/LConn1 -- v_a+/RConn1 -- Controlled Current Source/LConn1
  Voltage Measurement/LConn2 -- Controlled Current Source/RConn1 -- v_a-/RConn1
  Voltage Measurement1/LConn1 -- v_b+/RConn1 -- Controlled Current Source1/LConn1
  Controlled Current Source1/RConn1 -- v_b-/RConn1 -- Voltage Measurement1/LConn2
  Controlled Current Source2/LConn1 -- v_c+/RConn1 -- Voltage Measurement2/LConn1
  Voltage Measurement2/LConn2 -- v_c-/RConn1 -- Controlled Current Source2/RConn1

== system RTInductionMotorJan27/Motor Model/first test (g results with simscape but without feedback)/Electromagnetic Torque ==
  i_ds : Inport
  i_qs : Inport  Port=2
  P : Inport  Port=3
  Constant : Constant  Value=3/4
  Product{,1..3} (4 alike) : Product
  Subtract : Sum  Inputs=+-
  Te : Outport  VectorParamsAs1DForOutWhenUnconnected=off
  tag scope: Te=global
  wires:
  Product3/1 -> Te/1, [Te]
  Subtract/1 -> Product3/1
  Product2/1 -> Product3/2
  Constant/1 -> Product2/2
  P/1 -> Product2/1
  Product1/1 -> Subtract/2
  Product/1 -> Subtract/1
  i_ds/1 -> Product1/2
  [flux_qr] -> Product1/1
  [flux_dr] -> Product/2
  i_qs/1 -> Product/1

== system RTInductionMotorJan27/Motor Model/first test (g results with simscape but without feedback)/Rotor current ==
  Rr : Inport
  Lr : Inport  Port=2
  Lm : Inport  Port=3
  w_s : Inport  Port=4
  w_r : Inport  Port=5
  Rotor Flux : Subsystem
  Rotor currents : Subsystem
  Subtract : Sum  Inputs=+-
  i_dr : Outport  VectorParamsAs1DForOutWhenUnconnected=off
  i_qr : Outport  Port=2  VectorParamsAs1DForOutWhenUnconnected=off
  wires:
  Subtract/1 -> Rotor Flux/2(w_s1)
  w_r/1 -> Subtract/2
  w_s/1 -> Subtract/1
  Rotor currents/2(i_qr) -> i_qr/1
  Rotor currents/1(i_dr) -> i_dr/1
  Lm/1 -> Rotor currents/4(Lm)
  Lr/1 -> Rotor currents/3(Lr)
  Rr/1 -> Rotor Flux/1(Rr (Ohms))
  Rotor Flux/1(flux_dr) -> Rotor currents/1(flux_dr)  "flux_dr"
  Rotor Flux/2(flux_qr) -> Rotor currents/2(flus_qr)  "flux_qr"

== system RTInductionMotorJan27/Motor Model/first test (g results with simscape but without feedback)/Rotor speed ==
  J : Inport
  Divide : Product  Inputs=*/
  Integrator : Integrator
  Subtract : Sum  Inputs=+--
  TL : Constant  Value=0
  w_r : Outport  VectorParamsAs1DForOutWhenUnconnected=off
  wires:
  Integrator/1 -> w_r/1, Subtract/3
  Divide/1 -> Integrator/1
  J/1 -> Divide/2
  Subtract/1 -> Divide/1
  TL/1 -> Subtract/2
  [Te] -> Subtract/1

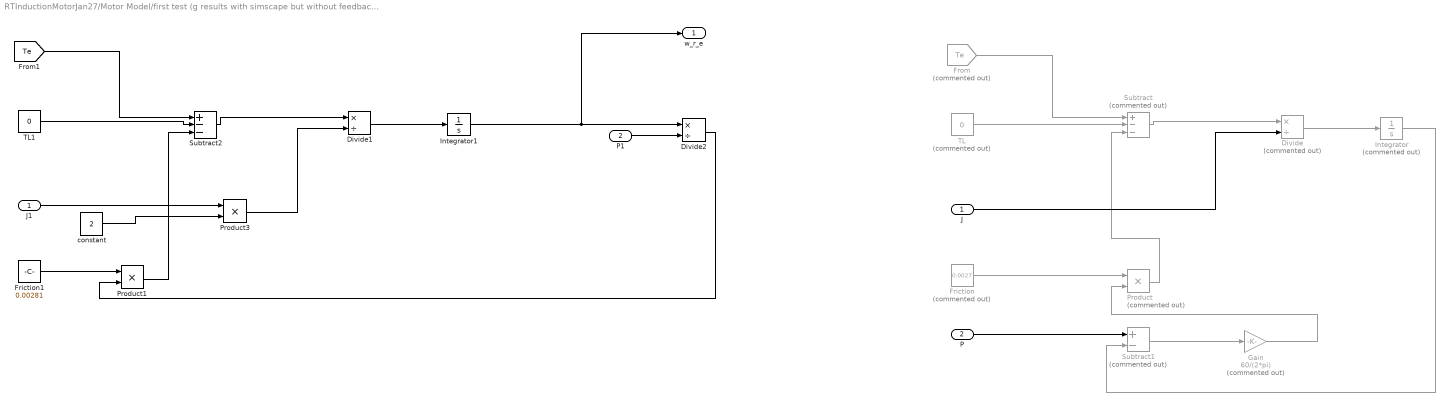
== system RTInductionMotorJan27/Motor Model/first test (g results with simscape but without feedback)/Rotor speed1 ==
  J : Inport
  P : Inport  Port=2
  Divide : Product  Commented=on  Inputs=*/
  Divide1 : Product  Inputs=*/
  Divide2 : Product  Inputs=*/
  Friction : Constant  Commented=on  Value=0.0027
  Friction1 : Constant  Value=0.00281
  From : From  Commented=on  GotoTag=Te  TagVisibility=global
  Gain : Gain  Commented=on  Gain=60/(2*pi)
  Integrator : Integrator  Commented=on
  Integrator1 : Integrator
  J1 : InportShadow
  P1 : InportShadow  Port=2
  Product : Product  Commented=on
  Product1 : Product
  Product3 : Product
  Subtract : Sum  Commented=on  Inputs=+--
  Subtract1 : Sum  Commented=on  Inputs=+-
  Subtract2 : Sum  Inputs=+--
  TL : Constant  Commented=on  Value=0
  TL1 : Constant  Value=0
  constant : Constant  Value=2
  w_r_e : Outport  VectorParamsAs1DForOutWhenUnconnected=off
  wires:
  Divide2/1 -> Product1/2
  P1/1 -> Divide2/2
  Integrator1/1 -> Divide2/1, w_r_e/1
  Product3/1 -> Divide1/2
  constant/1 -> Product3/2
  J1/1 -> Product3/1
  Product1/1 -> Subtract2/3
  Friction1/1 -> Product1/1
  TL1/1 -> Subtract2/2
  Divide1/1 -> Integrator1/1
  Subtract2/1 -> Divide1/1
  [Te] -> Subtract2/1
  Product/1 -> Subtract/3
  Friction/1 -> Product/1
  Gain/1 -> Product/2
  Subtract1/1 -> Gain/1
  P/1 -> Subtract1/1
  Integrator/1 -> Subtract1/2
  Divide/1 -> Integrator/1
  J/1 -> Divide/2
  Subtract/1 -> Divide/1
  TL/1 -> Subtract/2
  From/1 -> Subtract/1

== system RTInductionMotorJan27/Motor Model/first test (g results with simscape but without feedback)/Stator current ==
  Rs : Inport
  Ls : Inport  Port=2
  Lm : Inport  Port=3
  w_s : Inport  Port=4
  dq0 : Inport  Port=5
  Stator Flux : Subsystem
  Stator currents : Subsystem
  i_ds : Outport  VectorParamsAs1DForOutWhenUnconnected=off
  i_qs : Outport  Port=2  VectorParamsAs1DForOutWhenUnconnected=off
  wires:
  dq0/1 -> Stator Flux/3(dq0)
  Stator currents/2(i_qs) -> i_qs/1
  w_s/1 -> Stator Flux/2(w_s)
  Stator currents/1(i_ds) -> i_ds/1
  Lm/1 -> Stator currents/4(Lm)
  Ls/1 -> Stator currents/3(Ls)
  Rs/1 -> Stator Flux/1(Rs (Ohms))
  Stator Flux/1(flux_ds) -> Stator currents/1(flus_ds)  "flux_ds"
  Stator Flux/2(flux_qs) -> Stator currents/2(flus_qs)  "flux_qs"

== system RTInductionMotorJan27/Motor Model/first test (g results with simscape but without feedback)/dq ==
  P : Inport
  Demux1 : Demux  Outputs=3
  Mux : Mux  Inputs=3
  Scope : Scope  NumInputPorts=3
  Subsystem : Subsystem
  Voltage Measurement : powerlib/Measurements/Voltage Measurement  PhasorSimulation=off  OutputType=Complex  PSBequivalent=0
  Voltage Measurement1 : powerlib/Measurements/Voltage Measurement  PhasorSimulation=off  OutputType=Complex  PSBequivalent=0
  Voltage Measurement2 : powerlib/Measurements/Voltage Measurement  PhasorSimulation=off  OutputType=Complex  PSBequivalent=0
  abc to dq0 : powerlib_meascontrol/Transformations/abc to dq0  Alignment=90 degrees behind phase A axis
  v_a+ : PMIOPort  Side=Left
  v_a- : PMIOPort  Port=2  Side=Left
  v_b+ : PMIOPort  Port=3  Side=Left
  v_b- : PMIOPort  Port=4  Side=Left
  v_c+ : PMIOPort  Port=5  Side=Left
  v_c- : PMIOPort  Port=6  Side=Left
  dq0 : Outport  VectorParamsAs1DForOutWhenUnconnected=off
  wires:
  Demux1/3 -> Scope/3
  Demux1/2 -> Scope/2
  Demux1/1 -> Scope/1
  abc to dq0/1 -> dq0/1, Demux1/1
  Subsystem/1(w_t) -> abc to dq0/2
  P/1 -> Subsystem/1(P)
  Mux/1 -> abc to dq0/1
  Voltage Measurement2/1 -> Mux/3
  Voltage Measurement1/1 -> Mux/2
  Voltage Measurement/1 -> Mux/1
  connections:
  Voltage Measurement2/LConn2 -- v_c-/RConn1
  v_c+/RConn1 -- Voltage Measurement2/LConn1
  v_b-/RConn1 -- Voltage Measurement1/LConn2
  Voltage Measurement1/LConn1 -- v_b+/RConn1
  Voltage Measurement/LConn2 -- v_a-/RConn1
  Voltage Measurement/LConn1 -- v_a+/RConn1

== system RTInductionMotorJan27/Motor Model/test/Induction Machine ==
  Motor Parameters : Inport
  TL (Nm) : Inport  Port=2
  Frictional Torque (N.m.s) : Inport  Port=3
  Constant : Constant  Value=120
  Demux : Demux  Outputs=2
  Demux2 : Demux  Outputs=5
  EM Torque : Subsystem
  Fluxes to Currents : Subsystem
  Freq : Constant  Value=60
  Rotor Flux : Subsystem
  Rotor Speed : Subsystem
  Scope1 : Scope  NumInputPorts=2
  Stator Flux : Subsystem
  V_ll : Constant  Value=200
  abc : Subsystem
  abc-dq : Subsystem
  ns (rpm) : Product  Inputs=**/
  v_m : Gain  Gain=sqrt(2)/sqrt(3)
  w_s : Gain  Gain=2*pi/60
  EM Torque (Nm) : Outport  VectorParamsAs1DForOutWhenUnconnected=off
  wires:
  abc-dq/1(dq) -> Demux/1, Stator Flux/3(V_s dq0)  "Vs dq0"
  Rotor Flux/1(Phi_r dq) -> Fluxes to Currents/2(Phi_r dq)  "Phi_r dq"
  Fluxes to Currents/1(i_s dq) -> EM Torque/1(I_s dq), Stator Flux/1(I_s dq)  "i_s dq"
  Fluxes to Currents/2(i_r dq) -> EM Torque/2(I_r dq), Rotor Flux/3(I_r dq)  "i_r dq"
  Demux/1 -> Scope1/1  "Vs_d"
  Stator Flux/1(Phi_s dq) -> Fluxes to Currents/1(Phi_s dq)  "Phi_s dq"
  TL (Nm)/1 -> Rotor Speed/3(Load Torque (N))  "Load Torque (Nm)"
  EM Torque/1(EM Torque) -> Rotor Speed/1(EM Torque (N)), EM Torque (Nm)/1  "EM Torque (Nm)"
  Demux2/4 -> ns (rpm)/3, Rotor Speed/4(Pole Pairs), EM Torque/4(P)  "P"
  Demux/2 -> Scope1/2  "Vs_q"
  Rotor Speed/2(omega_r_e (rads-1)) -> Rotor Flux/1(omega_r)
  Frictional Torque (N.m.s)/1 -> Rotor Speed/2(Friction (N.m.s))
  Demux2/1 -> EM Torque/3(Lm), Fluxes to Currents/3(Lm)  "Lm"
  Demux2/2 -> Fluxes to Currents/4(Llr)  "Llr"
  Demux2/3 -> Fluxes to Currents/5(Lls)  "Lls"
  Motor Parameters/1 -> Demux2/1
  Demux2/5 -> Rotor Speed/5(Shaft Innertia (kg . m2))  "J"
  V_ll/1 -> v_m/1
  v_m/1 -> abc/1(Vm)
  ns (rpm)/1 -> w_s/1
  Freq/1 -> ns (rpm)/1
  Constant/1 -> ns (rpm)/2
  abc/1(v_a) -> abc-dq/4(v_a)
  abc/2(v_c) -> abc-dq/2(v_c)
  abc/3(v_b) -> abc-dq/1(v_b)
  w_s/1 -> Rotor Flux/2(omega_s), Stator Flux/2(omega_s), abc-dq/3(w_s)  "w_s"

== system RTInductionMotorJan27/Motor Model/test/Induction Motor Parameters1 ==
  Llr (H) : Constant  Value=30e-3
  Lls (H) : Constant  Value=30e-3
  Lm (H) : Constant  Value=0.495
  Mux : Mux  Inputs=5
  Pole Pairs : Constant  Value=4
  Rotor Inertia (kg.m2) : Constant  Value=0.011787
  Induction Motor Paramaters : Outport  VectorParamsAs1DForOutWhenUnconnected=off
  wires:
  Rotor Inertia (kg.m2)/1 -> Mux/5
  Mux/1 -> Induction Motor Paramaters/1
  Lm (H)/1 -> Mux/1
  Pole Pairs/1 -> Mux/4
  Llr (H)/1 -> Mux/3
  Lls (H)/1 -> Mux/2

== system RTInductionMotorJan27/Motor Model/test/Induction Motor Parameters2 ==
  Lm (H) : Constant  Value=0.0538
  Lr (H) : Constant  Value=0.056
  Ls (H) : Constant  Value=0.0553
  Mux : Mux  Inputs=5
  Pole Pairs : Constant  Value=4
  Rotor Inertia (kg.m2) : Constant  Value=0.0165
  Induction Motor Paramaters : Outport  VectorParamsAs1DForOutWhenUnconnected=off
  wires:
  Rotor Inertia (kg.m2)/1 -> Mux/5
  Mux/1 -> Induction Motor Paramaters/1
  Lm (H)/1 -> Mux/1
  Pole Pairs/1 -> Mux/4
  Lr (H)/1 -> Mux/3
  Ls (H)/1 -> Mux/2

== system RTInductionMotorJan27/Motor Model/first test (g results with feedback and simscape)/Rotor current/Rotor Flux ==
  Rr (Ohms) : Inport
  w_s1 : Inport  Port=2
  Integrator : Integrator
  Integrator1 : Integrator
  Rr (Ohms)1 : InportShadow
  Subtract : Sum  Inputs=-+
  Subtract1 : Sum  Inputs=--
  product{,1..3} (4 alike) : Product  Inputs=**
  flux_dr : Outport  VectorParamsAs1DForOutWhenUnconnected=off
  flux_qr : Outport  Port=2  VectorParamsAs1DForOutWhenUnconnected=off
  tag scope: flux_dr=global, flux_qr=global
  wires:
  Rr (Ohms)/1 -> product/2
  product/1 -> Subtract/1
  Subtract/1 -> Integrator/1
  Integrator/1 -> product2/1, [flux_dr], flux_dr/1
  Subtract1/1 -> Integrator1/1
  product1/1 -> Subtract1/2
  [i_dr] -> product/1
  Integrator1/1 -> product3/2, [flux_qr], flux_qr/1
  Rr (Ohms)1/1 -> product1/1
  w_s1/1 -> product3/1, product2/2
  product3/1 -> Subtract/2
  product2/1 -> Subtract1/1
  [i_qr] -> product1/2

== system RTInductionMotorJan27/Motor Model/first test (g results with feedback and simscape)/Rotor current/Rotor currents ==
  flux_dr : Inport
  flus_qr : Inport  Port=2
  Lr : Inport  Port=3
  Lm : Inport  Port=4
  Add : Sum
  Divide : Product  Inputs=*/
  Divide1 : Product  Inputs=/*
  Lm1 : InportShadow  Port=4
  Product : Product
  Product1 : Product
  Scope : Scope  NumInputPorts=2
  Subtract : Sum  Inputs=-+
  Subtract1 : Sum  Inputs=-+
  i_dr : Outport  VectorParamsAs1DForOutWhenUnconnected=off
  i_qr : Outport  Port=2  VectorParamsAs1DForOutWhenUnconnected=off
  tag scope: i_dr=global, i_qr=global
  wires:
  Lm1/1 -> Product/1
  [i_ds] -> Product/2
  flux_dr/1 -> Subtract/2
  Product/1 -> Subtract/1
  Lr/1 -> Add/1
  Lm/1 -> Product1/1, Add/2
  Subtract/1 -> Divide/1
  Add/1 -> Divide1/1, Divide/2
  Divide/1 -> [i_dr], Scope/2, i_dr/1  "i_dr"
  [i_qs] -> Product1/2
  Product1/1 -> Subtract1/1
  flus_qr/1 -> Subtract1/2
  Subtract1/1 -> Divide1/2
  Divide1/1 -> [i_qr], Scope/1, i_qr/1  "i_rs"

== system RTInductionMotorJan27/Motor Model/first test (g results with feedback and simscape)/Stator current/Stator Flux ==
  Rs (Ohms) : Inport
  w_s : Inport  Port=2
  dq0 : Inport  Port=3
  Demux : Demux  Outputs=3
  Integrator : Integrator
  Integrator1 : Integrator
  Rs (Ohms)1 : InportShadow
  Scope : Scope  NumInputPorts=2
  Subtract : Sum  Inputs=-++
  Subtract1 : Sum  Inputs=-+-
  Terminator : Terminator
  product{,1..3} (4 alike) : Product  Inputs=**
  w_s1 : InportShadow  Port=2
  flux_ds : Outport  VectorParamsAs1DForOutWhenUnconnected=off
  flux_qs : Outport  Port=2  VectorParamsAs1DForOutWhenUnconnected=off
  wires:
  dq0/1 -> Demux/1
  Rs (Ohms)/1 -> product/2
  product/1 -> Subtract/1  "i_ds*R_s"
  Subtract/1 -> Integrator/1
  Integrator/1 -> product2/1, Scope/1, flux_ds/1  "flux_ds"
  Subtract1/1 -> Integrator1/1
  product1/1 -> Subtract1/3
  [i_ds] -> product/1
  Integrator1/1 -> product3/2, Scope/2, flux_qs/1  "flux_qs"
  Rs (Ohms)1/1 -> product1/1
  w_s1/1 -> product3/1
  product3/1 -> Subtract/3
  w_s/1 -> product2/2
  product2/1 -> Subtract1/1
  [i_qs] -> product1/2
  Demux/1 -> Subtract/2  "v_ds"
  Demux/2 -> Subtract1/2  "v_qs"
  Demux/3 -> Terminator/1

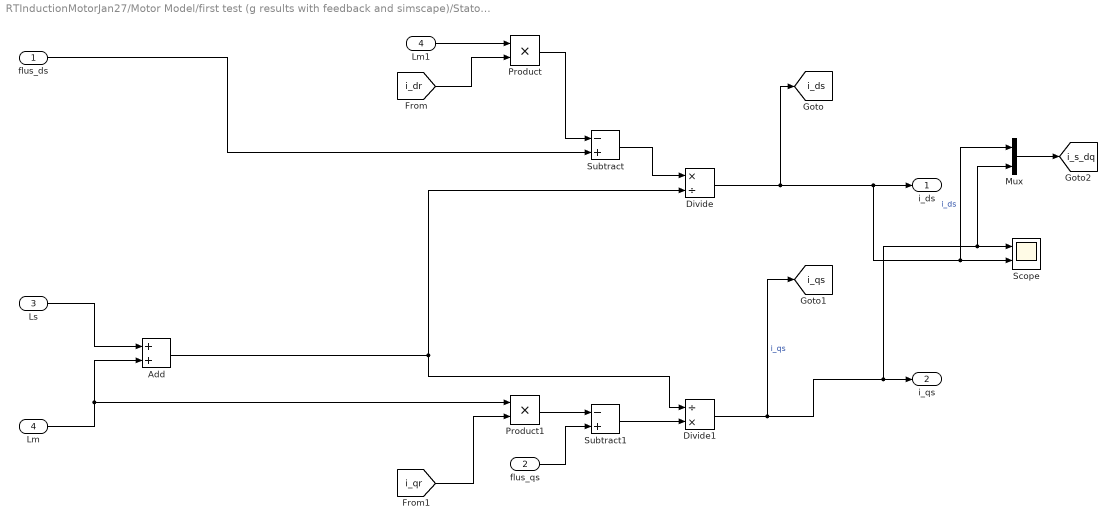
== system RTInductionMotorJan27/Motor Model/first test (g results with feedback and simscape)/Stator current/Stator currents ==
  flus_ds : Inport
  flus_qs : Inport  Port=2
  Ls : Inport  Port=3
  Lm : Inport  Port=4
  Add : Sum
  Divide : Product  Inputs=*/
  Divide1 : Product  Inputs=/*
  Lm1 : InportShadow  Port=4
  Mux : Mux  Inputs=2
  Product : Product
  Product1 : Product
  Scope : Scope  NumInputPorts=2
  Subtract : Sum  Inputs=-+
  Subtract1 : Sum  Inputs=-+
  i_ds : Outport  VectorParamsAs1DForOutWhenUnconnected=off
  i_qs : Outport  Port=2  VectorParamsAs1DForOutWhenUnconnected=off
  tag scope: i_ds=global, i_qs=global, i_s_dq=global
  wires:
  Lm1/1 -> Product/1
  [i_dr] -> Product/2
  flus_ds/1 -> Subtract/2
  Product/1 -> Subtract/1
  Ls/1 -> Add/1
  Lm/1 -> Product1/1, Add/2
  Subtract/1 -> Divide/1
  Add/1 -> Divide1/1, Divide/2
  Divide/1 -> [i_ds], Mux/1, Scope/2, i_ds/1  "i_ds"
  [i_qr] -> Product1/2
  Product1/1 -> Subtract1/1
  flus_qs/1 -> Subtract1/2
  Subtract1/1 -> Divide1/2
  Divide1/1 -> [i_qs], Mux/2, Scope/1, i_qs/1  "i_qs"
  Mux/1 -> [i_s_dq]
